simulink model "sample_model"  (R2023a)
settings: Solver=FixedStepAuto  StartTime=0.0  StopTime=10.0  RelTol=1e-3
undefined symbols (not defined in the file): Data_Display, untitled
libraries: androidsensorlib x2, androidaudiovideolib x2, androiduilib x1
settings Model: Creator=ragha  LastModifiedBy=ragha
settings OptimizationCC: EnhancedBackFolding=on  PassReuseOutputArgsAs=Individual arguments  ZeroExternalMemoryAtStartup=off  ZeroInternalMemoryAtStartup=off  MaxStackSize=64  OptimizeBlockOrder=speed  DifferentSizesBufferReuse=on  OptimizationCustomize=off  EfficientTunableParamExpr=on
settings DebuggingCC: ParameterTunabilityLossMsg=error
settings HardwareCC: ProdBitPerPointer=32  ProdBitPerSizeT=32  ProdBitPerPtrDiffT=32  ProdLargestAtomicInteger=Long  ProdLargestAtomicFloat=Double  ProdWordSize=32  ProdHWDeviceType=ARM Compatible->ARM Cortex
settings SFSimCC: MATLABDynamicMemAlloc=off
settings RTWCC: Description=Embedded Coder  SystemTargetFile=ert.tlc  HardwareBoard=Android Device  TLCOptions="-aInlineSetEventsForThisBaseRateFcn=TLC_FALSE -aSuppressMultiTaskScheduler=TLC_FALSE  -aRateBasedStepFcn=0"  TemplateMakefile=ert_default_tmf  RTWVerbose=off  Toolchain=Android SDK/NDK Tools
settings CodeAppCC: ForceParamTrailComments=on  IgnoreCustomStorageClasses=off  OperatorAnnotations=on  SimulinkDataObjDesc=on  SFDataObjDesc=on  InsertBlockDesc=on

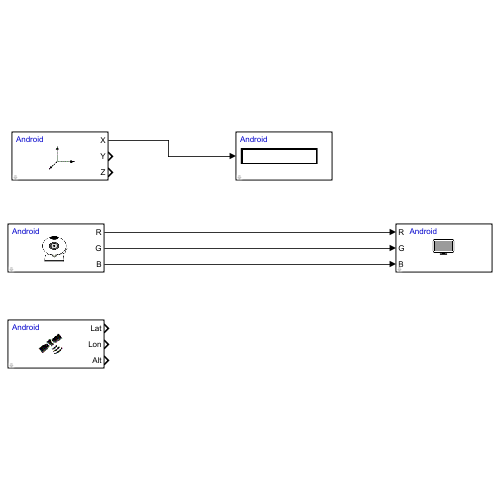
[thumbnail: Simulink's stored preview of the top-level diagram]
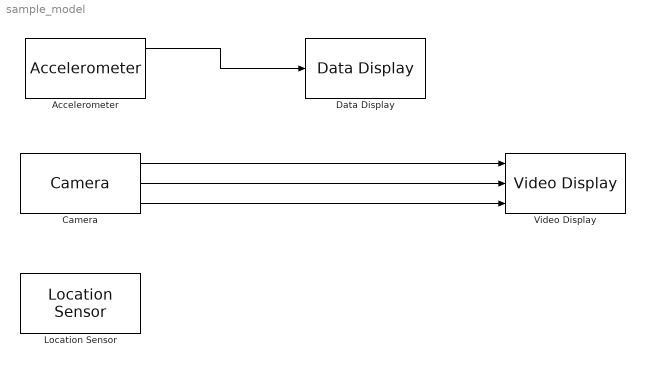
== system sample_model ==
  Accelerometer : androidsensorlib/Accelerometer  OutputVector=off  SampleTime=0.1  BlockPlatform=Android
  Camera : androidaudiovideolib/Camera  CameraLocation=Back  CameraResolutions=Back - 640x480  Width=640  Height=480  SampleTime=0.1  BlockPlatform=Android
  Data Display : androiduilib/Data Display  DataDisplayId=untitled/Data_Display  Format=Float  Precision=6  SimulateUsing=Code generation  blockPlatform=Android
  Location Sensor : androidsensorlib/Location Sensor  OutputVector=off  SampleTime=0.1  BlockPlatform=Android
  Video Display : androidaudiovideolib/Video Display  BlockPlatform=Android
  wires:
  Camera/1 -> Video Display/1
  Camera/2 -> Video Display/2
  Camera/3 -> Video Display/3
  Accelerometer/1 -> Data Display/1
